simulink model "X_Nucleo_IHM03A1"  (R2015a)
settings: Solver=FixedStepDiscrete  SolverMode=SingleTasking  StartTime=0.0  StopTime=10.0  FixedStep=1e-3  RelTol=1e-3
libraries: mbed_targets_stm_nucleo_f446 x1, mbed_spi_power x1, mbed_lib x1
settings Model: Creator=oh  LastModifiedBy=oh
settings OptimizationCC: OptimizeModelRefInitCode=on  LifeSpan=1
settings HardwareCC: ProdLargestAtomicInteger=Long  ProdLargestAtomicFloat=Double  ProdEndianess=LittleEndian  ProdHWDeviceType=ARM Compatible->ARM Cortex
settings RTWCC: SystemTargetFile=mbed.tlc  TemplateMakefile=mbed.tmf  Description=Mbed Target (Embedded Target)  TargetLang=C++
settings CodeAppCC: IgnoreCustomStorageClasses=off
settings STFCustomTargetCC: CombineOutputUpdateFcns=on  SupportContinuousTime=off  SupportVariableSizeSignals=off  SystemTargetFile=mbed.tlc
settings ERTTargetCC: SupportContinuousTime=off  SupportVariableSizeSignals=off  ERTCustomFileTemplate=mbed_file_process.tlc

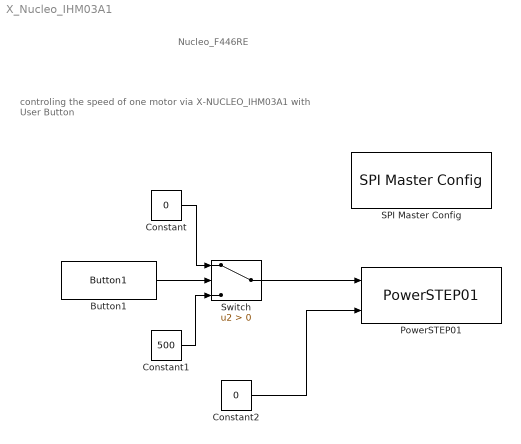
== system X_Nucleo_IHM03A1 ==
  note: Nucleo_F446RE
  note: controling the speed of one motor
      | via X-NUCLEO_IHM03A1 with User Button
  Button1 : mbed_targets_stm_nucleo_f446/Button1  Parameter1=0
  Constant : Constant  Value=0  OutDataTypeStr=uint32
  Constant1 : Constant  Value=500  OutDataTypeStr=uint32
  Constant2 : Constant  Value=0  OutDataTypeStr=uint8
  PowerSTEP01 : mbed_spi_power/PowerSTEP01  SpiPort=1  CsPort=B  CsPin=6  RstPort=A  RstPin=9  Cmd=Move  NumMotors=1  Acc=10000  Dec=10000  MaxSpd=1000  MinSpd=0  StepMode_=1/4 Step  Voltage_real=70
  SPI Master Config : mbed_lib/SPI/SPI Master Config  Priority=0  SpiPort=1  SpiFreq=100000  MosiPort=A  MosiPin=7  MisoPort=A  MisoPin=6  SclkPort=A  SclkPin=5
  Switch : Switch  Criteria=u2 > Threshold  OutDataTypeStr=Inherit: Inherit via back propagation
  wires:
  Button1/1 -> Switch/2
  Constant/1 -> Switch/1
  Constant1/1 -> Switch/3
  Switch/1 -> PowerSTEP01/1
  Constant2/1 -> PowerSTEP01/2
